simulink model "xEMU_SimulationModel3_rule1"  (R2017b)
settings: Solver=ode4  StartTime=0.0  StopTime=8192  FixedStep=0.01  RelTol=1e-3
undefined symbols (not defined in the file): a1, a2, a3, a4, ACO, BAT, Battery, DCT, DRT, EMS, ENV, Fahrzyklus_VS_modell, height_BAT, leistung, lib_bat, Maximum, Maximum_position, Num_cells, P_FC_max_long, P_FC_min_long, P_FC_step_max, Pbat_charge_max, Pbat_discharge_max, Pfc_max, Pfc_min, SOC_tar, time_peaks, TRM, velocity_peaks
libraries: simulink x5
(part 15 of 15)

== system xEMU_SimulationModel3_rule1/Battery (BAT)_mittel_02/Cell/ElectricalCircuit/SerialTwoPort_Elem1/Cellelement_Elem1/ParallelRC_Elem2 ==
  T : Inport
  SoC : Inport  Port=2
  Object : Lookup_n-D  BreakpointsForDimension1=[10 25 35 45]  BreakpointsForDimension2=[0 1 2 3 4 5 6 7 8 9 10 11 12 13 14 15 16 17 18 19 20 21 22 23 24 25 26 27 28 29 30 31 32 33 34 35 36 37 38 39 40 41 42 43 44 45 46 47 48 49 50 51 52 53 54 55 56 57 58 59 60 61 62 63 64 65 66 67 68 69 70 71 72 73 74 75 76 77 78 79 80 81 82 83 84 85 86 87 88 89 90 91 92 93 94 95 96 97 98 99 100]  Table=[0.0013859 0.0013859 0.0013859 0.0013859 0.0013859 0.0013859 0.0013926 0.0013992 0.0014058 0.0014123 0.0012987 0.0011812 0.0010627 0.0009443 0.00082615 0.00071478 0.00068406 0.00065311 0.00062216 0.00059122 0.00056306 0.00054867 0.00053424 0.00051981 0.00050538 0.00049175 0.00047966 0.00046745 0.00045518 0.00044285 0.000433 0.00042804 0.0004231 0.00041817 0.00041324 0.0004081 0.0004023 0.00039647 0.00039067 0.00038489 0.00037995 0.0003777 0.00037546 0.0003732 0.00037094 0.00036852 0.00036506 0.00036148 0.00035795 0.00035445 0.00035136 0.00035548 0.00035964 0.00036378 0.00036791 0.00037202 0.00038514 0.00040062 0.00041608 0.00043152 0.00044694 0.00046542 0.00048599 0.00050655 0.00052711 0.00054768 0.00056824 0.00058951 0.0006112 0.00061133 0.00060533 0.00059934 0.00059338 0.00056073 0.00052332 0.00048592 0.00044832 0.00044181 0.00043626 0.00043071 0.00042518 0.00041944 0.00041163 0.0004038 0.00039593 0.00038804 0.0003805 0.00038123 0.00038197 0.00038271 0.00038345 0.00038436 0.00038905 0.00039373 0.00039841 0.0004031 0.00041011 0.00042494 0.00043976 0.00045457 0.00046939;0.0013909 0.0013909 0.0013909 0.0013909 0.0013909 0.0013909 0.0012677 0.0011442 0.0010201 0.00089531 0.00076987 0.00070813 0.00067092 0.00063387 0.00059698 0.00056024 0.00054071 0.00052609 0.00051146 0.0004968 0.00048212 0.00047083 0.00046001 0.00044923 0.00043847 0.00042776 0.00042441 0.00042247 0.00042052 0.00041856 0.00041661 0.00041317 0.00040953 0.00040589 0.00040225 0.00039862 0.00040004 0.00040205 0.00040406 0.00040607 0.00040808 0.0004092 0.00040999 0.00041078 0.00041157 0.00041236 0.0004215 0.00043357 0.00044563 0.00045769 0.00046975 0.00047997 0.00048931 0.00049866 0.000508 0.00051734 0.00052631 0.00053508 0.00054384 0.00055261 0.00056137 0.00057128 0.00058201 0.00059273 0.00060345 0.00061444 0.00062577 0.00062186 0.00060878 0.00059619 0.00058364 0.00057119 0.00055875 0.00054632 0.00053389 0.00052147 0.00051268 0.00051153 0.00051035 0.00050914 0.00050791 0.00050053 0.00048201 0.00046349 0.00044497 0.00042644 0.00041137 0.00041072 0.00041006 0.0004094 0.00040874 0.00040944 0.00041633 0.00042321 0.00043009 0.00043696 0.00044609 0.00046351 0.00048093 0.00049835 0.00051577;0.00077991 0.00078732 0.00079473 0.0008022 0.00080973 0.00081733 0.00077298 0.00072439 0.0006758 0.00062721 0.00057863 0.00053152 0.00051203 0.00049254 0.00047306 0.00045358 0.00043529 0.00042495 0.00041461 0.00040427 0.00039392 0.00038532 0.00038231 0.00037931 0.0003763 0.0003733 0.0003706 0.00036924 0.00036788 0.00036654 0.00036521 0.0003638 0.00036211 0.00036043 0.00035874 0.00035706 0.00035728 0.00036183 0.00036638 0.00037093 0.00037548 0.00038001 0.00038438 0.00038876 0.00039314 0.00039752 0.00040459 0.00041569 0.00042679 0.00043789 0.00044899 0.00045895 0.00046692 0.00047489 0.00048286 0.00049083 0.00049744 0.00050096 0.00050448 0.000508 0.00051152 0.00051749 0.00052694 0.00053677 0.00054945 0.00055678 0.00055656 0.00055508 0.00054938 0.00053409 0.00051883 0.00050361 0.00048843 0.00047327 0.00045816 0.00044308 0.0004303 0.00042175 0.00041321 0.00040466 0.00039612 0.00039148 0.00039393 0.00039638 0.00039883 0.00040127 0.00040362 0.00040531 0.00040698 0.00040864 0.00041028 0.00041152 0.0004095 0.00040751 0.00040553 0.00040357 0.00040364 0.00041919 0.00043473 0.00045026 0.00046579;0.0012855 0.0011625 0.0010393 0.00091519 0.00079 0.00066376 0.00056433 0.00053552 0.00050663 0.00047766 0.00044861 0.0004226 0.00041044 0.00039826 0.00038604 0.0003738 0.00036359 0.00035862 0.00035368 0.00034876 0.00034387 0.00033958 0.0003363 0.00033301 0.00032972 0.00032644 0.00032545 0.00032681 0.00032819 0.00032958 0.00033097 0.00033077 0.00032916 0.00032756 0.00032595 0.00032434 0.00032735 0.00033368 0.00034002 0.00034635 0.00035268 0.00035828 0.00036341 0.00036854 0.00037368 0.00037881 0.00038558 0.00039298 0.00040038 0.00040778 0.00041518 0.0004202 0.00042445 0.00042871 0.00043296 0.00043721 0.00043943 0.00044019 0.00044094 0.00044168 0.0004424 0.00045681 0.00047378 0.00048444 0.00045479 0.0004251 0.00039518 0.00038272 0.00038064 0.00037803 0.00037546 0.00037292 0.00037041 0.00036793 0.00036548 0.00036306 0.00036395 0.00036685 0.00036974 0.00037264 0.00037553 0.00037697 0.00037675 0.00037652 0.00037628 0.00037602 0.00037578 0.00037567 0.00037556 0.00037545 0.00037536 0.00037505 0.00037108 0.00036709 0.0003631 0.0003591 0.00035518 0.00036521 0.00037569 0.00038619 0.00039667]  ExtrapMethod=Clip  RndMeth=Simplest  InputSameDT=on
  Tau : Lookup_n-D  BreakpointsForDimension1=[10 25 35 45]  BreakpointsForDimension2=[0 1 2 3 4 5 6 7 8 9 10 11 12 13 14 15 16 17 18 19 20 21 22 23 24 25 26 27 28 29 30 31 32 33 34 35 36 37 38 39 40 41 42 43 44 45 46 47 48 49 50 51 52 53 54 55 56 57 58 59 60 61 62 63 64 65 66 67 68 69 70 71 72 73 74 75 76 77 78 79 80 81 82 83 84 85 86 87 88 89 90 91 92 93 94 95 96 97 98 99 100]  Table=[6.9609 6.9609 6.9609 6.9609 6.9609 6.9609 6.8714 6.7814 6.6906 6.5993 7.9017 8.8824 9.5213 9.8203 9.7807 9.4733 9.8384 10.133 10.3575 10.5119 10.609 10.7316 10.834 10.9156 10.9764 11.0007 10.9688 10.9229 10.8636 10.7908 10.7399 10.7563 10.7704 10.7813 10.7889 10.7721 10.7052 10.6355 10.5638 10.4902 10.4359 10.4526 10.4694 10.4853 10.5002 10.5312 10.6222 10.7069 10.7884 10.8667 10.9438 11.0623 11.1821 11.3015 11.4207 11.5395 11.821 12.1335 12.433 12.7195 12.993 13.3494 13.7554 14.146 14.521 14.8805 15.2244 15.5661 15.8989 15.8496 15.6947 15.5399 15.3856 14.7348 13.9669 13.1684 12.3331 12.1622 12.0124 11.8629 11.7138 11.5629 11.3823 11.1999 11.0158 10.8299 10.6504 10.649 10.6475 10.6459 10.6442 10.6455 10.7112 10.7755 10.8382 10.8993 10.98 11.1195 11.2409 11.3441 11.4295;7.4878 7.4878 7.4878 7.4878 7.4878 7.4878 8.8506 9.8154 10.3811 10.5438 10.2997 10.4207 10.7112 10.9105 11.0194 11.0386 11.1802 11.3514 11.496 11.6139 11.705 11.7504 11.776 11.7885 11.7877 11.7739 11.8788 12.0097 12.1392 12.2673 12.3938 12.4095 12.4099 12.4083 12.4047 12.3992 12.5063 12.6277 12.7497 12.8724 12.9956 13.0468 13.0737 13.1007 13.1277 13.1547 13.3485 13.5947 13.8333 14.0643 14.2878 14.4344 14.5399 14.6388 14.731 14.8164 14.8932 14.9644 15.0299 15.0895 15.1434 15.2302 15.3391 15.4411 15.5361 15.6311 15.7276 15.5634 15.2408 14.9119 14.586 14.2684 13.9505 13.6325 13.3144 12.9963 12.7814 12.7851 12.7885 12.7916 12.7943 12.6984 12.4134 12.1142 11.8008 11.4731 11.1987 11.2003 11.2019 11.2034 11.2047 11.2225 11.3154 11.4052 11.4917 11.5749 11.6777 11.8533 12.0078 12.1412 12.2536;8.5561 8.5494 8.5409 8.5306 8.5185 8.5046 9.1102 9.5571 9.8673 10.0408 10.0775 9.9973 10.1881 10.3366 10.4426 10.5062 10.543 10.652 10.7435 10.8175 10.874 10.9348 11.0547 11.1713 11.2847 11.3949 11.4914 11.5519 11.6116 11.6707 11.7292 11.769 11.7701 11.7707 11.7708 11.7705 11.8131 11.9538 12.0942 12.2344 12.3744 12.4989 12.5765 12.6525 12.7271 12.8001 12.9161 13.0912 13.2568 13.4128 13.5592 13.67 13.7274 13.7787 13.8238 13.8628 13.869 13.8115 13.7517 13.6899 13.6258 13.6061 13.6388 13.6706 13.7358 13.6556 13.3857 13.075 12.7762 12.5714 12.359 12.1391 11.9116 11.6766 11.4342 11.1842 10.9946 10.917 10.8337 10.7447 10.65 10.6311 10.758 10.8856 11.014 11.1432 11.2651 11.3374 11.4096 11.4815 11.5533 11.6119 11.5617 11.5118 11.4622 11.413 11.3779 11.4389 11.472 11.4771 11.4542;6.4369 7.9789 9.0676 9.7014 9.8688 9.558 9.1358 9.3851 9.5559 9.6481 9.6613 9.6399 9.7752 9.8854 9.9706 10.0304 10.0967 10.2309 10.3582 10.4784 10.5918 10.6822 10.7478 10.8102 10.8692 10.9249 10.9893 11.0644 11.1399 11.2158 11.2921 11.3191 11.3021 11.2847 11.2671 11.2491 11.3466 11.5264 11.7047 11.8815 12.0568 12.1598 12.2145 12.2658 12.3138 12.3584 12.42 12.4842 12.5419 12.593 12.6375 12.6074 12.5515 12.4919 12.4286 12.3616 12.2497 12.1068 11.9629 11.818 11.6721 11.6591 11.6433 11.5078 10.7923 10.076 9.355 9.1544 9.2689 9.3814 9.4925 9.6021 9.7103 9.8171 9.9226 10.0269 10.1379 10.2579 10.3785 10.4997 10.6216 10.6982 10.7213 10.744 10.7662 10.788 10.8102 10.8372 10.8644 10.8917 10.9192 10.9399 10.8428 10.745 10.6468 10.5479 10.4493 10.4148 10.3638 10.2941 10.2048]  ExtrapMethod=Clip  RndMeth=Simplest  InputSameDT=on
  tag scope: ID4_ObjR=global, ID4_ObjTau=global
  wires:
  Object/1 -> [ID4_ObjR]
  T/1 -> Object/1, Tau/1
  SoC/1 -> Object/2, Tau/2
  Tau/1 -> [ID4_ObjTau]

== system xEMU_SimulationModel3_rule1/Battery (BAT)_mittel_02/Cell/ElectricalCircuit/SerialTwoPort_Elem1/Cellelement_Elem1/ParallelRC_Elem3 ==
  T : Inport
  SoC : Inport  Port=2
  Object : Lookup_n-D  BreakpointsForDimension1=[10 25 35 45]  BreakpointsForDimension2=[0 1 2 3 4 5 6 7 8 9 10 11 12 13 14 15 16 17 18 19 20 21 22 23 24 25 26 27 28 29 30 31 32 33 34 35 36 37 38 39 40 41 42 43 44 45 46 47 48 49 50 51 52 53 54 55 56 57 58 59 60 61 62 63 64 65 66 67 68 69 70 71 72 73 74 75 76 77 78 79 80 81 82 83 84 85 86 87 88 89 90 91 92 93 94 95 96 97 98 99 100]  Table=[0.0023581 0.0023581 0.0023581 0.0023581 0.0023581 0.0023581 0.0023667 0.0023751 0.0023836 0.002392 0.0022544 0.0021111 0.0019664 0.0018219 0.0016777 0.0015413 0.001498 0.0014543 0.0014105 0.0013668 0.001328 0.0013132 0.0012983 0.0012835 0.0012686 0.0012573 0.0012546 0.0012519 0.0012493 0.0012467 0.0012445 0.0012429 0.0012413 0.0012397 0.001238 0.0012371 0.0012377 0.0012383 0.0012388 0.0012393 0.0012404 0.0012434 0.0012466 0.0012497 0.0012529 0.0012538 0.0012458 0.0012379 0.0012299 0.0012219 0.0012142 0.0012128 0.0012112 0.0012096 0.001208 0.0012065 0.0012145 0.0012247 0.0012349 0.0012451 0.0012553 0.0013094 0.0013929 0.0014764 0.0015599 0.0016433 0.0017268 0.0018186 0.0019153 0.0019239 0.0019056 0.0018818 0.0018581 0.0017177 0.0015565 0.0013953 0.0012339 0.0011999 0.0011697 0.0011397 0.0011097 0.0010817 0.0010647 0.0010478 0.001031 0.0010142 0.00099788 0.00098791 0.00097792 0.00096791 0.00095789 0.00094784 0.00093761 0.00092737 0.00091714 0.00090691 0.00090393 0.00092541 0.00094689 0.00096837 0.00098971;0.0018533 0.0018533 0.0018533 0.0018533 0.0018533 0.0018533 0.0016946 0.0015355 0.0013757 0.001215 0.0010534 0.00097611 0.00093055 0.00088526 0.00084026 0.00079553 0.00078111 0.00077554 0.00076996 0.00076437 0.00075875 0.00075966 0.00076183 0.00076399 0.00076616 0.00076832 0.00076457 0.00075989 0.0007552 0.00075051 0.00074582 0.00074345 0.00074135 0.00073926 0.00073717 0.00073507 0.00073237 0.00072953 0.00072668 0.00072383 0.00072098 0.00071511 0.00070852 0.00070194 0.00069535 0.00068876 0.00067879 0.00066747 0.00065616 0.00064484 0.00063352 0.00062673 0.0006222 0.00061766 0.00061312 0.00060858 0.00061444 0.00062865 0.00064285 0.00065706 0.00067126 0.00073495 0.00083615 0.00093717 0.001038 0.0011429 0.0012528 0.0011804 0.00099463 0.00080227 0.00065744 0.00063071 0.00060385 0.00057685 0.00054972 0.00052245 0.00050089 0.00049146 0.00048206 0.00047267 0.00046331 0.00045896 0.00046373 0.0004685 0.00047327 0.00047804 0.00048123 0.00047775 0.00047427 0.00047079 0.00046731 0.00046352 0.00045821 0.0004529 0.00044759 0.00044228 0.00044251 0.00046378 0.00048506 0.00050633 0.00052761;0.00098803 0.00099419 0.0010004 0.0010066 0.0010129 0.0010192 0.00095902 0.00089542 0.00083183 0.00076825 0.00070468 0.00064369 0.00063007 0.00061646 0.00060284 0.00058923 0.0005772 0.00057523 0.00057326 0.00057129 0.00056932 0.00056827 0.0005701 0.00057194 0.00057378 0.00057561 0.0005758 0.00057087 0.00056596 0.00056107 0.00055619 0.00055183 0.00054834 0.00054486 0.00054139 0.00053793 0.00053493 0.00053289 0.00053086 0.00052882 0.00052678 0.00052167 0.00050858 0.0004955 0.00048242 0.00046934 0.0004577 0.00044812 0.00043853 0.00042895 0.00041936 0.00041089 0.00040479 0.00039869 0.00039258 0.00038648 0.00038703 0.00040216 0.00041728 0.00043241 0.00044754 0.00048353 0.00054305 0.00060302 0.00066462 0.00064251 0.000506 0.00036892 0.00027022 0.00027969 0.00028913 0.00029854 0.00030791 0.00031726 0.00032657 0.00033584 0.00034025 0.00033587 0.00033149 0.00032711 0.00032273 0.00031716 0.00030948 0.0003018 0.00029412 0.00028644 0.00027913 0.00027418 0.00026924 0.00026433 0.00025944 0.0002549 0.00025322 0.00025154 0.00024986 0.00024818 0.00024849 0.00026379 0.00027904 0.00029431 0.00030957;0.0012377 0.0011354 0.0010326 0.00092905 0.00082461 0.00071928 0.00063436 0.00060577 0.00057704 0.00054816 0.00051915 0.000494 0.00048711 0.00048019 0.00047323 0.00046626 0.00046033 0.00045733 0.00045432 0.00045132 0.00044831 0.00044496 0.00044121 0.00043746 0.00043371 0.00042996 0.0004278 0.00042706 0.00042635 0.00042565 0.00042498 0.00042194 0.00041687 0.00041181 0.00040676 0.00040171 0.00039681 0.00039203 0.00038725 0.00038248 0.0003777 0.00037026 0.00036089 0.00035152 0.00034215 0.00033278 0.00032263 0.00031234 0.00030204 0.00029175 0.00028146 0.00027911 0.00027918 0.00027925 0.00027933 0.0002794 0.00028345 0.00029059 0.0002977 0.00030478 0.00031182 0.00031848 0.00032622 0.00033143 0.00031812 0.00030067 0.00027662 0.00026056 0.00025208 0.00024984 0.00024757 0.00024527 0.00024294 0.00024058 0.0002382 0.00023578 0.00022957 0.00022093 0.00021229 0.00020365 0.00019501 0.00018831 0.00018396 0.00017962 0.0001753 0.00017098 0.00016691 0.00016423 0.00016153 0.00015884 0.00015613 0.00015347 0.00015169 0.00014991 0.00014813 0.00014635 0.00014465 0.00016237 0.00018065 0.00019892 0.00021712]  ExtrapMethod=Clip  RndMeth=Simplest  InputSameDT=on
  Tau : Lookup_n-D  BreakpointsForDimension1=[10 25 35 45]  BreakpointsForDimension2=[0 1 2 3 4 5 6 7 8 9 10 11 12 13 14 15 16 17 18 19 20 21 22 23 24 25 26 27 28 29 30 31 32 33 34 35 36 37 38 39 40 41 42 43 44 45 46 47 48 49 50 51 52 53 54 55 56 57 58 59 60 61 62 63 64 65 66 67 68 69 70 71 72 73 74 75 76 77 78 79 80 81 82 83 84 85 86 87 88 89 90 91 92 93 94 95 96 97 98 99 100]  Table=[54.8457 54.8457 54.8457 54.8457 54.8457 54.8457 54.3726 53.8976 53.4206 52.9416 53.8148 54.3677 54.4193 53.9261 52.8888 51.5133 52.4112 53.1852 53.8206 54.3176 54.7002 55.194 55.6763 56.1335 56.5654 56.7527 56.3792 55.9963 55.6104 55.2214 54.9745 55.0602 55.1517 55.2402 55.3259 55.2877 54.9533 54.6122 54.2726 53.9346 53.6109 53.3672 53.1377 52.908 52.678 52.3975 51.7771 51.119 50.4745 49.8433 49.2501 49.1884 49.1314 49.0686 49.0003 48.9262 50.0867 51.6121 53.1528 54.7088 56.28 59.4967 63.881 68.3367 72.864 77.463 82.1339 86.8362 91.5326 90.3877 87.5608 84.665 81.7986 74.1421 65.8794 57.8881 50.1322 48.842 47.7481 46.6581 45.5712 44.6471 44.1255 43.5861 43.0295 42.4566 41.8696 41.8655 41.8502 41.8239 41.7865 41.7417 41.931 42.1063 42.2677 42.4151 42.8105 44.1193 45.451 46.8063 48.1919;59.5282 59.5282 59.5282 59.5282 59.5282 59.5282 63.0384 64.8951 65.1034 63.6499 60.5212 59.3153 59.2027 58.8348 58.2162 57.3512 57.4466 57.8947 58.3345 58.766 59.189 59.1391 58.9495 58.7602 58.5712 58.3826 58.3145 58.2816 58.2447 58.204 58.1593 57.6398 57.0758 56.5141 55.9546 55.3974 55.3694 55.3658 55.3606 55.3537 55.3451 54.6878 53.8379 52.9943 52.1572 51.3266 51.7183 52.4264 53.0813 53.6829 54.2313 54.8238 55.4641 56.0892 56.6993 57.2942 58.3016 59.7581 61.2196 62.686 64.1572 68.6373 74.7687 80.061 84.5102 87.1453 87.2726 80.5288 70.034 59.9204 51.5267 50.744 49.8685 48.8955 47.8204 46.6384 45.9889 46.6315 47.2046 47.7093 48.1464 47.6926 45.6783 43.6125 41.4949 39.3257 37.5631 37.6732 37.7764 37.8728 37.9624 38.1949 39.1505 40.0733 40.9631 41.8202 42.6856 43.6155 44.4425 45.1665 45.7875;64.1531 63.8467 63.5295 63.2008 62.8603 62.5076 63.3508 63.7471 63.4905 62.5813 61.0196 58.9218 58.415 57.8762 57.3052 56.7022 56.0827 55.612 55.1431 54.676 54.2108 53.9522 54.3285 54.7061 55.085 55.4652 55.6623 55.3759 55.0917 54.8097 54.5299 54.1531 53.5309 52.9129 52.2993 51.6898 51.4035 51.9131 52.4174 52.9163 53.4098 53.5386 52.6907 51.8174 50.9186 49.9944 49.9462 51.2551 52.4632 53.5706 54.5773 55.47 56.2021 56.8874 57.5257 58.1171 58.7537 59.259 59.6307 59.8688 59.9734 61.3035 63.4275 64.3508 63.8779 69.5339 76.5767 71.7864 60.3652 59.1998 57.8156 56.2147 54.3992 52.3711 50.1327 47.6859 45.2159 43.168 41.1583 39.1868 37.2536 36.2935 36.9767 37.5821 38.1098 38.5598 39.0395 40.1293 41.1661 42.1498 43.0802 43.82 43.4647 43.132 42.8218 42.5342 42.5547 44.7519 46.8957 48.9898 51.0337;53.3106 62.307 68.9198 73.1198 74.8458 74.0347 71.4012 69.9387 68.2988 66.4798 64.4798 62.4499 61.1408 59.8448 58.5617 57.2915 56.3043 55.9913 55.6782 55.365 55.0517 54.5757 53.8883 53.2048 52.5251 51.8494 51.8739 52.5748 53.278 53.9837 54.692 54.5509 53.674 52.8035 51.9392 51.0812 51.4674 52.6946 53.8769 55.0141 56.1064 56.5354 56.4692 56.3322 56.1243 55.8455 56.6307 57.6211 58.4271 59.0487 59.486 60.1106 60.8322 61.5542 62.2765 62.9991 62.307 60.595 58.7059 56.6402 54.3983 54.05 54.1679 54.15 53.2608 51.9014 49.6907 48.1457 47.34 47.0934 46.8457 46.5968 46.3462 46.0938 45.8392 45.5822 46.2292 47.1948 47.9487 48.491 48.8217 48.9975 49.1534 49.2533 49.2973 49.2858 49.3496 50.1763 50.9454 51.6569 52.3107 52.7663 50.7072 48.6768 46.6752 44.7026 42.7808 45.6476 48.1324 50.0896 51.5202]  ExtrapMethod=Clip  RndMeth=Simplest  InputSameDT=on
  tag scope: ID5_ObjR=global, ID5_ObjTau=global
  wires:
  Object/1 -> [ID5_ObjR]
  T/1 -> Object/1, Tau/1
  SoC/1 -> Object/2, Tau/2
  Tau/1 -> [ID5_ObjTau]

== system xEMU_SimulationModel3_rule1/Battery (BAT)_mittel_02/Cell/ElectricalCircuit/SerialTwoPort_Elem1/Cellelement_Elem1/VoltageSource_Elem5 ==
  T : Inport
  SoC : Inport  Port=2
  Object : Lookup_n-D  BreakpointsForDimension1=[10 25 35 45]  BreakpointsForDimension2=[0 1 2 3 4 5 6 7 8 9 10 11 12 13 14 15 16 17 18 19 20 21 22 23 24 25 26 27 28 29 30 31 32 33 34 35 36 37 38 39 40 41 42 43 44 45 46 47 48 49 50 51 52 53 54 55 56 57 58 59 60 61 62 63 64 65 66 67 68 69 70 71 72 73 74 75 76 77 78 79 80 81 82 83 84 85 86 87 88 89 90 91 92 93 94 95 96 97 98 99 100]  Table=[2.051 2.0595 2.0672 2.0736 2.0794 2.0847 2.0897 2.0946 2.0994 2.1039 2.1084 2.1127 2.117 2.1211 2.1251 2.1291 2.133 2.1368 2.1404 2.144 2.1476 2.151 2.1544 2.1576 2.1608 2.1638 2.1669 2.1699 2.1729 2.1759 2.1789 2.1819 2.1848 2.1878 2.1908 2.1938 2.1968 2.1999 2.2032 2.2066 2.2102 2.2138 2.2175 2.2215 2.2257 2.23 2.2343 2.2388 2.2435 2.2485 2.2536 2.2588 2.2641 2.2698 2.2759 2.2821 2.2885 2.295 2.3018 2.3087 2.3155 2.322 2.3279 2.3322 2.3352 2.3378 2.34 2.342 2.3439 2.3453 2.3466 2.3481 2.3504 2.3547 2.3591 2.3637 2.3688 2.3749 2.3814 2.3875 2.3936 2.3999 2.4065 2.4136 2.4202 2.427 2.4342 2.4423 2.4506 2.4583 2.4658 2.4736 2.4822 2.4912 2.4996 2.5079 2.5165 2.5256 2.5371 2.5532 2.5734;2.051 2.0595 2.0672 2.0736 2.0794 2.0847 2.0897 2.0946 2.0994 2.1039 2.1084 2.1127 2.117 2.1211 2.1251 2.1291 2.133 2.1368 2.1404 2.144 2.1476 2.151 2.1544 2.1576 2.1608 2.1638 2.1669 2.1699 2.1729 2.1759 2.1789 2.1819 2.1848 2.1878 2.1908 2.1938 2.1968 2.1999 2.2032 2.2066 2.2102 2.2138 2.2175 2.2215 2.2257 2.23 2.2343 2.2388 2.2435 2.2485 2.2536 2.2588 2.2641 2.2698 2.2759 2.2821 2.2885 2.295 2.3018 2.3087 2.3155 2.322 2.3279 2.3322 2.3352 2.3378 2.34 2.342 2.3439 2.3453 2.3466 2.3481 2.3504 2.3547 2.3591 2.3637 2.3688 2.3749 2.3814 2.3875 2.3936 2.3999 2.4065 2.4136 2.4202 2.427 2.4342 2.4423 2.4506 2.4583 2.4658 2.4736 2.4822 2.4912 2.4996 2.5079 2.5165 2.5256 2.5371 2.5532 2.5734;2.051 2.0595 2.0672 2.0736 2.0794 2.0847 2.0897 2.0946 2.0994 2.1039 2.1084 2.1127 2.117 2.1211 2.1251 2.1291 2.133 2.1368 2.1404 2.144 2.1476 2.151 2.1544 2.1576 2.1608 2.1638 2.1669 2.1699 2.1729 2.1759 2.1789 2.1819 2.1848 2.1878 2.1908 2.1938 2.1968 2.1999 2.2032 2.2066 2.2102 2.2138 2.2175 2.2215 2.2257 2.23 2.2343 2.2388 2.2435 2.2485 2.2536 2.2588 2.2641 2.2698 2.2759 2.2821 2.2885 2.295 2.3018 2.3087 2.3155 2.322 2.3279 2.3322 2.3352 2.3378 2.34 2.342 2.3439 2.3453 2.3466 2.3481 2.3504 2.3547 2.3591 2.3637 2.3688 2.3749 2.3814 2.3875 2.3936 2.3999 2.4065 2.4136 2.4202 2.427 2.4342 2.4423 2.4506 2.4583 2.4658 2.4736 2.4822 2.4912 2.4996 2.5079 2.5165 2.5256 2.5371 2.5532 2.5734;2.051 2.0595 2.0672 2.0736 2.0794 2.0847 2.0897 2.0946 2.0994 2.1039 2.1084 2.1127 2.117 2.1211 2.1251 2.1291 2.133 2.1368 2.1404 2.144 2.1476 2.151 2.1544 2.1576 2.1608 2.1638 2.1669 2.1699 2.1729 2.1759 2.1789 2.1819 2.1848 2.1878 2.1908 2.1938 2.1968 2.1999 2.2032 2.2066 2.2102 2.2138 2.2175 2.2215 2.2257 2.23 2.2343 2.2388 2.2435 2.2485 2.2536 2.2588 2.2641 2.2698 2.2759 2.2821 2.2885 2.295 2.3018 2.3087 2.3155 2.322 2.3279 2.3322 2.3352 2.3378 2.34 2.342 2.3439 2.3453 2.3466 2.3481 2.3504 2.3547 2.3591 2.3637 2.3688 2.3749 2.3814 2.3875 2.3936 2.3999 2.4065 2.4136 2.4202 2.427 2.4342 2.4423 2.4506 2.4583 2.4658 2.4736 2.4822 2.4912 2.4996 2.5079 2.5165 2.5256 2.5371 2.5532 2.5734]  ExtrapMethod=Clip  RndMeth=Simplest  InputSameDT=on
  tag scope: ID6_ObjV=global
  wires:
  Object/1 -> [ID6_ObjV]
  T/1 -> Object/1
  SoC/1 -> Object/2

== system xEMU_SimulationModel3_rule1/Energy Manager (EMA)/Kern von EMS/P_load_aver/Subsystem/traction_motor_kennfeldbasiert/Subsystem ==
  M : Inport
  "lookuptable_Pv " : Inport  Port=2
  "n " : Inport  Port=3
  MATLAB Function : MATLAB Function  TreatAsAtomicUnit=on
  n-D Lookup Pv_obergrenze : Lookup_n-D  NumberOfTableDimensions=1  BreakpointsForDimension1=DRT.motor.speedvector  BreakpointsForDimension3=[5, 7]  Table=DRT.motor.Pv_obergrenze  InternalRulePriority=Speed  RndMeth=Simplest  InputSameDT=on
  n-D Lookup Pv_untergrenze : Lookup_n-D  NumberOfTableDimensions=1  BreakpointsForDimension1=DRT.motor.speedvector  BreakpointsForDimension3=[5, 7]  Table=DRT.motor.Pv_untergrenze  InternalRulePriority=Speed  RndMeth=Simplest  InputSameDT=on
  Pv_motor : Outport
  wires:
  "n "/1 -> n-D Lookup Pv_untergrenze/1, n-D Lookup Pv_obergrenze/1
  M/1 -> MATLAB Function/4(M)
  n-D Lookup Pv_untergrenze/1 -> MATLAB Function/3(Pv_min)
  n-D Lookup Pv_obergrenze/1 -> MATLAB Function/2(Pv_max)
  "lookuptable_Pv "/1 -> MATLAB Function/1(Pv)
  MATLAB Function/1(y) -> Pv_motor/1

== matlab function xEMU_SimulationModel3_rule1/Energy Manager (EMA)/Umrechnung von Leistung auf Kraft2/MATLAB Function1 ==
  data: F_motor_durch_P input; F_motor_nach_EMS output; v input; v_soll input; F_motor_direkt input; F_driver input; F_brake_M_durch_P input; F_mech_nach_EMS output
function [F_motor_nach_EMS,F_mech_nach_EMS] = fcn(F_motor_durch_P,v, v_soll,F_motor_direkt, F_driver, F_brake_M_durch_P)
if v <= 1 && v >= 0
    F_motor_nach_EMS = F_motor_direkt;
    if F_driver >= 0
        F_mech_nach_EMS = 0;
    else
        F_mech_nach_EMS = F_driver - F_motor_direkt;
    end
else
    F_motor_nach_EMS = F_motor_durch_P;
    F_mech_nach_EMS = F_brake_M_durch_P;
end
% if v <= 0.005  && v_soll == 0
%    temp = F_motor_nach_EMS;
%    F_motor_nach_EMS = F_mech_nach_EMS;
%    F_mech_nach_EMS = temp;
% end

== matlab function xEMU_SimulationModel3_rule1/Energy Manager (EMA)/Kern von EMS/Subsystem/Ausschaltung der Batterie ==
  data: SoC input; P_bat output; Pbat input
function P_bat = fcn(SoC, Pbat)
P_bat = Pbat;
if SoC < 0.2 && Pbat > 0
    P_bat = 0;
end
if SoC> 0.9 && Pbat < 0
    P_bat = 0;
end

== matlab function xEMU_SimulationModel3_rule1/Drive Train (DRT)/Converter and traction motor/traction_motor_kennfeldbasiert/MATLAB Function1 ==
  data: M_soll input; M_min input; M_ist output; M_max input
function M_ist = fcn(M_soll,M_min, M_max)
if M_soll <= M_max && M_soll>= M_min
    M_ist = M_soll;
elseif M_soll > M_max
    M_ist = M_max;
else
    M_ist = M_min;
end

== matlab function xEMU_SimulationModel3_rule1/Energy Manager (EMA)/Umrechnung von Leistung auf Kraft/MATLAB Function ==
  data: u input; y output
function y = fcn(u)
if abs(u)< 0.001
    y = 0;
else
    y = u;
end

== matlab function xEMU_SimulationModel3_rule1/Energy Manager (EMA)/Umrechnung von Leistung auf Kraft/MATLAB Function1 ==
  data: u1 input; y output; u2 input
function y = fcn(u1,u2)
if abs(u1) < 10^-5
    y = 0;
else
    y = u1 / u2;
end

== matlab function xEMU_SimulationModel3_rule1/Energy Manager (EMA)/Kern von EMS/P_load_aver/Subsystem/traction_motor_kennfeldbasiert/MATLAB Function1 ==
  data: M_soll input; M_min input; M_ist output; M_max input
function M_ist = fcn(M_soll,M_min, M_max)
if M_soll <= M_max && M_soll>= M_min
    M_ist = M_soll;
elseif M_soll > M_max
    M_ist = M_max;
else
    M_ist = M_min;
end

== matlab function xEMU_SimulationModel3_rule1/Energy Manager (EMA)/Kern von EMS/P_load_aver/Subsystem/traction_motor_kennfeldbasiert/Subsystem/MATLAB Function ==
  data: Pv input; y output; Pv_max input; Pv_min input; M input
function y = fcn(Pv, Pv_max, Pv_min, M)
    if isnan(Pv)
        if M > 0 
            y = Pv_max;
        else
            y = Pv_min;
        end
    else
        y = Pv;
    end

== matlab function xEMU_SimulationModel3_rule1/Energy Manager (EMA)/Kern von EMS/P_load_aver/Subsystem/traction_motor_kennfeldbasiert/umrichter efficiency ==
  data: u input; y output
function y = fcn(u)
if u >0
    y = u/0.94;
else
    y = u*0.94;
end

== matlab function xEMU_SimulationModel3_rule1/Energy Manager (EMA)/Kern von EMS/P_load_aver/Subsystem/dcdc efficiency ==
  data: u input; y output
function y = fcn(u)
if u >0
    y = u/0.98;
else
    y = u*0.98;
end

== matlab function xEMU_SimulationModel3_rule1/Energy Manager (EMA)/Umrechnung von Leistung auf Kraft/MATLAB Function2 ==
  data: P_wunsch input; P_tractionDemand input; P_EMAdemand output; P_brakeMech output
function [P_EMAdemand,P_brakeMech] = fcn(P_wunsch,P_tractionDemand) 
    if P_wunsch>=0
        P_EMAdemand=P_tractionDemand;
        P_brakeMech=0;
    else
        P_EMAdemand=P_tractionDemand;
        P_brakeMech=P_wunsch-P_tractionDemand;
    end

== matlab function xEMU_SimulationModel3_rule1/Battery (BAT)_mittel/Battery/Thermal/ConductivityMatrix ==
  data: u input; y output
function y = fcn(u)
    y = ConductivityMatrix(u);
end

== matlab function xEMU_SimulationModel3_rule1/Battery (BAT)_komplex/Subsystem/Thermal/ConductivityMatrix ==
  data: u input; y output
function y = fcn(u)
    y = ConductivityMatrix(u);
end

== matlab function xEMU_SimulationModel3_rule1/Train Dynamics (TRM)/Variant Subsystem/v_s_model/Driving Resistances/MATLAB Function1 ==
  data: v input; froll input; Froll output
function Froll  = fcn(v,froll) 
    if v==0
        Froll=0;
%     else if v<1
%         Froll=froll*v;
    else
        Froll=froll;
    end

== matlab function xEMU_SimulationModel3_rule1/Battery (BAT)_mittel/Subsystem1/Thermal/ConductivityMatrix ==
  data: u input; y output
function y = fcn(u)
    y = ConductivityMatrix(u);
end

== matlab function xEMU_SimulationModel3_rule1/Battery (BAT)_mittel_02/Cell/Thermal/ConductivityMatrix ==
  data: u input; y output
function y = fcn(u)
    y = ConductivityMatrix(u);
end

== matlab function xEMU_SimulationModel3_rule1/Battery (BAT)_mittel_02/Cell/Thermal/Coolings/DefaultCooling_Elem1/DefaultCooling ==
  data: u input; y output; airTemperature input
function y = fcn(u, airTemperature)
    
y = DefaultCooling(u, airTemperature);

end

== matlab function xEMU_SimulationModel3_rule1/Train Dynamics (TRM)/Variant Subsystem/v_t_model/Driver1/MATLAB Function ==
  data: pid input; s output
function s = fcn(pid) 
    a=pid/100;
    if pid>=0
       s=a*21177*3*0.99;
    else
        s=a*21177*6*0.99;
    end

== matlab function xEMU_SimulationModel3_rule1/Drive Train (DRT)/gear efficiency ==
  data: t_motor input; t_axis output; data input
function t_axis = fcn(t_motor, data)

    if t_motor >= 0
        t_axis = data * t_motor;
        
    else 
        t_axis = t_motor/data;
        
    end

== matlab function xEMU_SimulationModel3_rule1/Train Dynamics (TRM)/Variant Subsystem/v_s_model/Driver1/MATLAB Function ==
  data: pid input; s output
function s = fcn(pid) 
    a=pid/100;
    if pid>=0
       s=a*21177*4*0.99;
    else s=a*21177*4*2*0.99;
    end

== matlab function xEMU_SimulationModel3_rule1/Train Dynamics (TRM)/Variant Subsystem/v_s_model/Driver1/MATLAB Function1 ==
  data: vsoll input; dv input; Reset output
function Reset = fcn(vsoll,dv) 
    if dv==0&&vsoll==0
        Reset=0;
    else
        Reset=1;
    end

== matlab function xEMU_SimulationModel3_rule1/DC Link Storage (DLS)/MATLAB Function ==
  data: t input; v_bat_average output; v_bat_total input
function v_bat_average = fcn(t, v_bat_total)
     
v_bat_average = v_bat_total/(t+0.1);

== matlab function xEMU_SimulationModel3_rule1/Battery (BAT)_komplex/MATLAB Function ==
  data: SOC_i input; Battery_consume_eff_rate output; I_bat input; Temp input
function Battery_consume_eff_rate = fcn(SOC_i, I_bat,Temp)
  
%      tmp1 = alpha_cal_matrix.*SOC_cal_matrix + beta_cal_matrix;
%      tmp2 = -31700+163.3*( abs(I_cal_matrix*Battery.n_parallel)/Battery.Capacity );
%      tmp3 = exp(tmp2./(Battery.R_const.*(Battery.Temp+273.15)));
%      
%      gamma_cal_matrix = (20/(tmp1.*tmp3)).^(1/0.57);
%      
%      theta_cal_matrix = Battery.life_nom/gamma_cal_matrix;
%      
%      Battery_consume_eff = theta_cal_matrix.*abs(I_cal_matrix*Battery.n_parallel)/Battery.lambda*delta_t;
%         
% 
% 
% 
    I_bat = abs(I_bat);
    alpha = 1.287600000000000e+03*(SOC_i<0.45)+ (SOC_i>=0.45)*1.385500000000000e+03;
    beta = 6.356300000000000e+03*(SOC_i<0.45) + (SOC_i>=0.45)*4.193200000000000e+03;
  
   % cauculate the battery life consumption
     tmp1 = alpha*SOC_i + beta;
     tmp2 = -31700+163.3*(I_bat/207);
     tmp3 = exp(tmp2/(8.314462618153240*(Temp+273.15)));
     
     gamma = (20/(tmp1*tmp3))^(1/0.57);
     
     theta = 149870/gamma;
     
     Battery_consume_eff_rate = theta*I_bat/3600;

== matlab function xEMU_SimulationModel3_rule1/Energy Manager (EMA)/Kern von EMS/P_load_aver/MATLAB Function3 ==
  data: SOC_tar input; P_load_aver_tmp input; SOC_current input; P_load_aver output; distance input; t input
function P_load_aver = fcn(SOC_tar, P_load_aver_tmp, SOC_current, distance, t)
if t>8192-600
    soc_diff = SOC_tar-SOC_current;
    P_load_aver_tmp = P_load_aver_tmp + soc_diff*(5000000/(154093 - distance));

    if P_load_aver_tmp>200
        P_load_aver_tmp =200;
    elseif P_load_aver_tmp<30
        P_load_aver_tmp=30;
    end
end
    P_load_aver = P_load_aver_tmp;

== matlab function xEMU_SimulationModel3_rule1/Fuel Cell System (FCS)/FC_system/MATLAB Function ==
  data: xx input; H2_consumption_gramspersec output; fuel_flow_2 parameter
function H2_consumption_gramspersec= fcn(xx,fuel_flow_2)
H2_consumption_gramspersec = interp1(0:200,fuel_flow_2,xx);



    
%H2_consumption_gramspersec=-4.753219174323936e-15.*(xx.^8)+2.002917435478188e-12.*(xx.^7)-3.418111194449961e-10.*(xx.^6)+3.048736741095524e-08.*(xx.^5)-1.533622376717681e-06.*(xx.^4)+4.416163371263360e-05.*(xx.^3)-6.623406928113584e-04.*(xx.^2)+0.019716069838035.*xx+0.012253824730904;
%H2_consumption_gramspersec=2*H2_consumption_gramspersec;

end

== matlab function xEMU_SimulationModel3_rule1/Train Dynamics (TRM)/Variant Subsystem/v_t_model/Driving Resistances/MATLAB Function1 ==
  data: v input; froll input; Froll output
function Froll  = fcn(v,froll) 
    if v==0
        Froll=0;
%     else if v<1
%         Froll=froll*v;
    else
        Froll=froll;
    end

== matlab function xEMU_SimulationModel3_rule1/Drive Train (DRT)/Converter and traction motor/traction_motor_kennfeldbasiert/Subsystem/MATLAB Function ==
  data: Pv input; y output; Pv_max input; Pv_min input; M input
function y = fcn(Pv, Pv_max, Pv_min, M)
    if isnan(Pv)
        if M > 0 
            y = Pv_max;
        else
            y = Pv_min;
        end
    else
        y = Pv;
    end

== matlab function xEMU_SimulationModel3_rule1/Drive Train (DRT)/Converter and traction motor/traction_motor_kennfeldbasiert/Subsystem1/MATLAB Function ==
  data: cosphi input; y output; cosphi_max input; cosphi_min input; M input
function y = fcn(cosphi, cosphi_max, cosphi_min, M)
    if isnan(cosphi)
        if M > 0 
            y = cosphi_max;
        else
            y = cosphi_min;
        end
    else
        y = cosphi;
    end

== matlab function xEMU_SimulationModel3_rule1/Energy Manager (EMA)/Kern von EMS/Leistungsflussverteilug /MATLAB Function1 ==
  data: P_load input; P_FCdemand_kW output; Mode input; SOC input; P_load_aver input; Pbat_charge_max parameter; Pfc_max parameter; Pbat_discharge_max parameter; a1 parameter; Pfc_min parameter
function P_FCdemand_kW = fcn(P_load, Mode, SOC, P_load_aver, Pbat_charge_max, Pfc_max, Pbat_discharge_max,a1,Pfc_min)
   

   buffer_auf = 50; %because there is a limit of the fuel cell power change rate,
                     %a buffer region is set up, so the fuel cell supply its maximal power
                     % before P_load = Pbat_max+Pfc_max, so the demanded power can be fulfilled
   buffer_ab = 0;   % analog, only to ensure there is less energy wasted
   P_FCdemand_kW = P_load_aver;
if Mode == 1
    if P_load > (Pbat_discharge_max + Pfc_max - buffer_auf)
        P_FCdemand_kW = Pfc_max;
        
    elseif P_load > (-Pbat_charge_max + buffer_ab)
        if SOC >= a1 - 0.08
            P_FCdemand_kW = P_load_aver + 60;
        elseif SOC< a1 - 0.08
            P_FCdemand_kW = P_load_aver + 100;
        end
        if SOC<= 0.2
            P_FCdemand_kW = Pfc_max; 
        end 
    else
        P_FCdemand_kW = Pfc_min;    
    end
    
elseif Mode == 2
    if P_load >= Pbat_discharge_max + Pfc_max - buffer_auf
        P_FCdemand_kW = Pfc_max;                    
    elseif P_load < Pbat_discharge_max + Pfc_max - buffer_auf&& P_load >= -Pbat_charge_max
        P_FCdemand_kW = P_load_aver;
    else
        P_FCdemand_kW = Pfc_min;     
    end
    
else % Mode ==3 
       if P_load >= Pbat_discharge_max + Pfc_max - buffer_auf
           P_FCdemand_kW = Pfc_max;
    
       elseif P_load >= (-Pbat_charge_max + buffer_ab)        
           P_FCdemand_kW = P_load_aver - 50;
           if SOC>=0.9
               P_FCdemand_kW = 0;
           end     
       else 
           P_FCdemand_kW = Pfc_min;
       end
end
 
% if P_FCdemand_kW > Pfc_max
%     P_FCdemand_kW = Pfc_max;
% elseif P_FCdemand_kW < Pfc_min
%     P_FCdemand_kW = Pfc_min;
% end

== matlab function xEMU_SimulationModel3_rule1/Energy Manager (EMA)/Kern von EMS/P_load_aver/P_load_aver ==
  data: height_bat input; height input; time input; peak_positions input; distance input; leistung input; v input; v_before input; P_Demand_aver_pred output; P_Demand_total input; t input; P_Demand_aver_before input; v_peak input
function P_Demand_aver_pred = fcn(height_bat, height, time,peak_positions,distance,leistung, v, v_before, P_Demand_total,t, P_Demand_aver_before, v_peak)

        if(v~=0 && v_before==0)
            P_Demand_aver_pred = P_Demand_total/(t+0.1);
            if t<300
               P_Demand_aver_pred = 100;
            end 
            %new method
                %i = 1;
                %for i = 1:length(peak_positions)
                    if distance < peak_positions(1)
                        P_Demand_aver_pred = P_Demand_aver_pred + (   60000 *9.81 * (height(1)-height_bat) + 0.5*60000* v_peak(1) * v_peak(1)  )/time(1)/1000  ;
                    else 
                        P_Demand_aver_pred = P_Demand_aver_pred - (   60000 *9.81 * (height(1)-height_bat) + 0.5*60000* v_peak(1) * v_peak(1)  )/(8193-time(1))/1000 ;
                    end
                %end
            %new method ends here
        else
            P_Demand_aver_pred = P_Demand_aver_before; 

        end
        if P_Demand_aver_pred>200
            P_Demand_aver_pred =200;
        elseif P_Demand_aver_pred<30
            P_Demand_aver_pred=30;
        end

== matlab function xEMU_SimulationModel3_rule1/Drive Train (DRT)/Converter and traction motor/traction_motor_kennfeldbasiert/Subsystem2/MATLAB Function ==
  data: U_LL input; y output; U_LL_max input; U_LL_min input; M input
function y = fcn(U_LL, U_LL_max, U_LL_min, M)
    if isnan(U_LL)
        if M > 0 
            y = U_LL_max;
        else
            y = U_LL_min;
        end
    else
        y = U_LL;
    end

== matlab function xEMU_SimulationModel3_rule1/Drive Train (DRT)/Converter and traction motor/traction_motor_kennfeldbasiert/Subsystem3/MATLAB Function ==
  data: I_strang input; y output; I_strang_max input; I_strang_min input; M input
function y = fcn(I_strang, I_strang_max, I_strang_min, M)
    if isnan(I_strang)
        if M > 0 
            y = I_strang_max;
        else
            y = I_strang_min;
        end
    else
        y = I_strang;
    end

== matlab function xEMU_SimulationModel3_rule1/Train Dynamics (TRM)/Variant Subsystem/v_t_model/Driver1/Subsystem/MATLAB Function1 ==
  data: M_soll input; M_min input; M_ist output; M_max input
function M_ist = fcn(M_soll,M_min, M_max)
if M_soll <= M_max && M_soll>= M_min
    M_ist = M_soll;
elseif M_soll > M_max
    M_ist = M_max;
else
    M_ist = M_min;
end

== matlab function xEMU_SimulationModel3_rule1/Train Dynamics (TRM)/Variant Subsystem/v_t_model/Driver1/Subsystem/MATLAB Function2 ==
  data: u input; F_em output; f_brake output
function [F_em, f_brake] = fcn(u)
f_brake = 0;

if u<-21177*3*0.99
    u = u + 21177*3*0.99;
    f_brake = -21177*3*0.99;
elseif u<0   
    f_brake = u;
    u = 0;
end

F_em = u;

== matlab function xEMU_SimulationModel3_rule1/Train Dynamics (TRM)/Variant Subsystem/v_t_model/Driver1/Subsystem/MATLAB Function3 ==
  data: f_soll input; f_actual output; f_can input
function f_actual = fcn(f_soll, f_can)

if abs(f_soll)>abs(f_can)
    f_soll = f_can;
end
f_actual = f_soll;

== matlab function xEMU_SimulationModel3_rule1/Drive Train (DRT)/Slipmodel and Traction /Variant Subsystem1/Mit_Schlupf_nach_Kalker/Tire Dynamics/MATLAB Function ==
  data: dv input; v input; s output
function s = fcn(dv,v) 
    s=dv/v
    end

== matlab function xEMU_SimulationModel3_rule1/Drive Train (DRT)/Slipmodel and Traction /Variant Subsystem1/Mit_Schlupf_nach_Kalker/Tire Dynamics/MATLAB Function1 ==
  data: wrad input; Mx input; Mrad output
function Mrad  = fcn(wrad,Mx) 
    if wrad<=0 && Mx<=0
        Mrad=0;
    else
        Mrad=Mx;
    end

== matlab function xEMU_SimulationModel3_rule1/Drive Train (DRT)/Slipmodel and Traction /Variant Subsystem1/Mit_Schlupf_nach_Yoshiki/Slip Model/MATLAB Function1 ==
  data: ad_factor input; ad_rail input; w input; v_ist input; v_soll input; ad_factor_final output
function ad_factor_final = fcn(ad_factor, ad_rail, w, v_ist, v_soll)
if v_soll == 0 &&v_ist>0 &&w==0
   ad_factor_final=-ad_rail;
else
   ad_factor_final=ad_factor;
end

== matlab function xEMU_SimulationModel3_rule1/Drive Train (DRT)/Slipmodel and Traction /Variant Subsystem1/Mit_Schlupf_nach_Yoshiki/Tire Dynamics/MATLAB Function ==
  data: dv input; v input; s output
function s = fcn(dv,v) 
    s=dv/v
    end

== matlab function xEMU_SimulationModel3_rule1/Drive Train (DRT)/Slipmodel and Traction /Variant Subsystem1/Mit_Schlupf_nach_Yoshiki/Tire Dynamics/MATLAB Function1 ==
  data: T_dem_per_axis input; v_soll input; T_dem_per_axis_final output
function T_dem_per_axis_final = fcn(T_dem_per_axis, v_soll)
if v_soll == 0
%if v_soll == 0 &&v_ist>0 &&w==0
   %T_dem_per_axis_final=T_dem_per_axis-0.3*60000*10/4/2*0.425
   T_dem_per_axis_final=T_dem_per_axis-10000
else
   T_dem_per_axis_final=T_dem_per_axis
end
